simulink library "tqd"  (R2021b)
settings: Solver=VariableStepAuto  StartTime=0.0  StopTime=10.0  RelTol=1e-3
undefined symbols (not defined in the file or in its folder): ATQD_APSDecReq_X_kph, ATQD_APSDecReq_Y_mps2, ATQD_APSDecReqCMD_X_kph, ATQD_APSDecReqTs_X_pct, ATQD_APSDecTimeGain_X_Deg, ATQD_APSDecTimeGain_Y_s, ATQD_APSReqLowSpd_X_Deg, ATQD_AutoHoldReleaseBPS_X_Deg, ATQD_AWDLoadTrqnsGain_X_kg, ATQD_AWDLoadTrqnsGain_Y_pct, ATQD_BOSEnBPSPosn_X_kph, ATQD_BOSMap_X_rpm, ATQD_BOSMap_Y_pct, ATQD_CreepBaseTqD_X_kph, ATQD_CreepBaseTqD_Y_Deg, ATQD_CreepBaseTqR_X_kph, ATQD_CreepBaseTqR_Y_Deg, ATQD_CreepBPSDisPosn_X_Deg, ATQD_CreepBPSDisPosnR_X_Deg, ATQD_CreepBPSEnPosn_X_Deg, ATQD_CreepBPSEnPosnR_X_Deg, ATQD_CreepDeltaTq_X_kph, ATQD_CreepIterm_X_kph, ATQD_CreepIterm_Y_kph, ATQD_CreepItermMaxLimit_X_pct, ATQD_CreepPreloadTime_X_kph, ATQD_CreepPreloadTq_X_kph, ATQD_CreepPreloadTq_Y_s, ATQD_CreepProtTq_X_Deg, ATQD_CreepPterm_X_kph, ATQD_ECOTqMapD_X_rpm, ATQD_ECOTqMapD_Y_pct, ATQD_EOPDTqMapDCon_X_rpm, ATQD_EOPDTqMapDCon_Y_Deg, ATQD_EstInitVehWeight_X_c, ATQD_LHMRollGenMapD_X_rpm, ATQD_LHMRollGenMapD_Y_rpm, ATQD_LHMTqMapD_X_rpm, ATQD_LHMTqMapD_Y_pct, ATQD_NL1TqMapD_X_rpm, ATQD_NL1TqMapD_Y_pct, ATQD_NOPDTqMapDCon_X_rpm, ATQD_NOPDTqMapDCon_Y_Deg, ATQD_NRMRrEDUSpRat_X_rpm, ATQD_NRMRrEDUSpRat_Y_Nm, ATQD_OPDHoldDownRelDelay_X_Deg, ATQD_OPDHoldEnSpd_X_Deg, ATQD_OPDHoldRelDetTime_X_Deg, ATQD_OPDHoldReleaseTq_X_Deg, ATQD_OrigPedTqLowLim_X_Deg, ATQD_OrigPedTqLowLim_Y_pct, ATQD_PedalMapClimbUpLim_X_rpm, ATQD_PedalMapClimbUpLim_Y_Deg, ATQD_PreLoadTq_X_s, ATQD_RollGenMapEL1_X_rpm, ATQD_RollGenMapEL1_Y_rpm, ATQD_SL1TqMapD_X_rpm, ATQD_SL1TqMapD_Y_pct, ATQD_SlideRegenTqGain_X_Gps, ATQD_SlideRegenTqGain_Y_pct ... (+378)
libraries: hcu_lib x59, simulink x49
(part 1 of 12)
settings Model: Creator=13615  LastModifiedBy=FVT22063
settings SolverCC: AlgebraicLoopSolver=TrustRegion
settings DataIOCC: SaveFormat=Array  SignalLoggingSaveFormat=ModelDataLogs  ReturnWorkspaceOutputs=off
settings OptimizationCC: BlockReduction=off  BooleanDataType=off
settings DebuggingCC: SaveWithParameterizedLinksMsg=none  UnderspecifiedInitializationDetection=Classic  MergeDetectMultiDrivingBlocksExec=none  SignalResolutionControl=TryResolveAllWithWarning
settings HardwareCC: TargetUnknown=on
settings ModelReferenceCC: PropagateSignalLabelsOutOfModel=off
settings SFSimCC: SimUseLocalCustomCode=off
settings RTWCC: RTWUseLocalCustomCode=off
settings ConfigComp: CovMetricSettings=dw  CovSaveCumulativeToWorkspaceVar=on  CovSaveSingleToWorkspaceVar=on

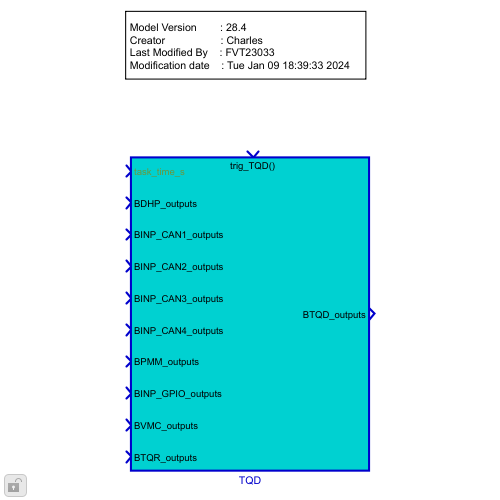
[thumbnail: Simulink's stored preview of the top-level diagram]
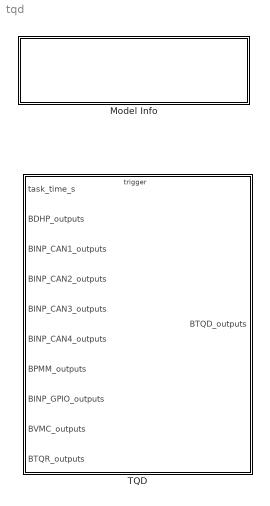
== system tqd ==
  Model Info : Subsystem  LoadFcn=slcm LoadBlock;  InitFcn=slcm('UpdateAllCMBlocksInThisModelInit')  mask(CMBlock){InitialSaveTempField=, InitialBlockCM=None, BlockCM=None, Frame=on, SaveTempField=, DisplayStringWithTags=|, MaskDisplayString=Model Version        : 26.218\nCreator                   : Charles\nLast Modified By    : FVT22063\nModification date    : Thu Sep 19 13:30:35 2024, HorizontalTextAlignment=Left, LeftAlignmentValue=0.02, SourceBlockDiagram=tqd, TagMaxNumber=20, CMTag1=, CMTag2=, CMTag3=, CMTag4=, CMTag5=, CMTag6=, CMTag7=, CMTag8=, CMTag9=, CMTag10=, CMTag11=, CMTag12=, CMTag13=, CMTag14=, CMTag15=, CMTag16=, CMTag17=, CMTag18=, CMTag19=, CMTag20=}
      mask DisplayStringWithTags=|
      | Model Version        : %<ModelVersion>
      | Creator                   : Charles
      | Last Modified By    : %<LastModifiedBy>
      | Modification date    : %<LastModificationDate>
      mask help: This block allows revision control information to be displayed within the model.
      settings: CopyFcn=slcm CopyBlock;  DeleteFcn=slcm Cancel;  PostSaveFcn=slcm('UpdateAllCMBlocksInThisModel')  NameChangeFcn=slcm Rename;  OpenFcn=slcm
      mask Display: text(str2num(LeftAlignmentValue), 0.5, MaskDisplayString, 'HorizontalAlignment', HorizontalTextAlignment)
  TQD : Subsystem
      settings: RTWSystemCode=Nonreusable function  RTWFcnNameOpts=Use subsystem name  RTWFileNameOpts=Use subsystem name

== system tqd/Model Info ==
  EmptySubsystem : Subsystem

== system tqd/TQD ==
  task_time_s : Inport
  BDHP_outputs : Inport  Port=2  OutDataTypeStr=Bus: BDHP_outputs
  BINP_CAN1_outputs : Inport  Port=3  OutDataTypeStr=Bus: BINP_CAN1_outputs
  BINP_CAN2_outputs : Inport  Port=4  OutDataTypeStr=Bus: BINP_CAN2_outputs
  BINP_CAN3_outputs : Inport  Port=5  OutDataTypeStr=Bus: BINP_CAN3_outputs
  BINP_CAN4_outputs : Inport  Port=6  OutDataTypeStr=Bus: BINP_CAN4_outputs
  BPMM_outputs : Inport  Port=7  OutDataTypeStr=Bus: BPMM_outputs
  BINP_GPIO_outputs : Inport  Port=8  OutDataTypeStr=Bus: BINP_GPIO_outputs
  BVMC_outputs : Inport  Port=9  OutDataTypeStr=Bus: BVMC_outputs
  BTQR_outputs : Inport  Port=10  OutDataTypeStr=Bus: BTQR_outputs  LockScale=on
  trig_TQD : TriggerPort  TriggerType=function-call  VariantControl=(inherit)
  Bus Creator1 : BusCreator  Inputs=78  OutDataTypeStr=Bus: BTQD_outputs  NonVirtualBus=on
  Bus Selector : BusSelector  OutputSignals=VINP_IVIPWModeReq_enum,VINP_IVICreepSWReq_flg,VINP_RollModeSWCmd_enum,VINP_IVIPwrLockSW_enum
  Bus Selector1 : BusSelector  OutputSignals=VDHP_ActAPSPosn_pct,VDHP_LowIdleAccPedal_flg
  Bus Selector2 : BusSelector  OutputSignals=VINP_VehSpeed_kph,VINP_BrkSwSta_flg,VINP_BrkSwV_flg,VINP_BrkPedalPos_pct,VINP_BrkPedalPosSta_flg,VINP_FrPTCSActive_flg,VINP_RrPTCSActive_flg,VINP_FrntAxlTrqReqDrv_Nm,VINP_RearAxlTrqReqDrv_Nm,VINP_FrRBCActive_flg,VINP_RrRBCActive_flg,VINP_FrntAxlTrqReqBrk_Nm,VINP_RearAxlTrqReqBrk_Nm,VINP_ADASForceIdle_flg,VINP_CrashOutputSts_enum,VINP_LongAccel_Gps,VINP_EPBCarWashMode_flg,VINP_EPBErrSta_enum,VINP_EPBSta_enum,VINP_DOASta_flg,VINP_HSAActive_flg,VINP_DriverSeatBeltCmd_flg,VINP_AVHActive_flg,VINP_ACCRequiredAccel_mps2,VINP_ACCVehHoldReq_flg,VINP_PsngrSeatBeltCmd_flg,VINP_RDriverSeatBeltCmd_flg,VINP_RCenterSeatBeltCmd_flg,VINP_RPsngrSeatBeltCmd_flg,VINP_SASAngle_Deg,VINP_YawRate_degps,VINP_ADASACCSta_enum,VINP_ABSActive_flg,VINP_ESCActive_flg
  Bus Selector3 : BusSelector  OutputSignals=VINP_BrakeSWGPIO_flg,VINP_CrashSignalGPIO_flg,VINP_DrDoorSW_flg,VINP_SeatSW_flg,VINP_HoodSW_flg,VINP_TailgateSW_flg,VINP_PsDoorSW_flg,VINP_RRDoorSW_flg,VINP_RLDoorSW_flg
  Bus Selector4 : BusSelector  OutputSignals=VINP_ShifterHandleCmd_enum,VINP_FrEDURotateDirction_enum,VINP_RrEDURotateDirction_enum,VINP_FrTMSpd_rpm,VINP_RrTMSpd_rpm,VINP_HVBPwrAvailDchrg_kW,VINP_HVBPwrAvailChrg_kW,VINP_FrRegenAvailTq_Nm,VINP_RrRegenAvailTq_Nm,VINP_FrEDURealTMTq_Nm,VINP_RrEDURealTMTq_Nm,VINP_HVBattErr_flg,VINP_DCDCFaultSta_enum,VINP_FrMotorAvailTq_Nm,VINP_RrMotorAvailTq_Nm,VINP_MCUWarnF_enum,VINP_MCUWarnR_enum,VINP_ChrgPlugSta_enum,VINP_HVBattSOC_pct
  Bus Selector5 : BusSelector  OutputSignals=VVMC_ADASActive_flg,VVMC_ADASWhlTqReq_Nm,VVMC_CruzActive_flg,VVMC_CruzWhlTqReq_Nm,VVMC_MSAActive_flg,VVMC_MSAWhlTqReq_Nm,VVMC_APSActive_flg,VVMC_APSSpeedCMD_kph,VVMC_APSShiftPosnReq_enum,VVMC_ACCPedalOvrd_flg,VVMC_LongAcc_Gps,VVMC_ActMaxSlideRate_pct,VVMC_EstSlope_Deg,VVMC_APSReq_enum,VVMC_RWDRDCActive_enum,VVMC_ActLRSlideRate_pct,VVMC_ActRRSlideRate_pct,VVMC_ActStESCYaw_Dps,VVMC_CAASActive_flg,VVMC_CalibratedGyroY_Dps
  Bus Selector6 : BusSelector  OutputSignals=VINP_RegenMode_enum,VINP_DrSCPSysErrLmp_flg
  Bus Selector7 : BusSelector  OutputSignals=VPMM_PowerSta_enum,VPMM_DrivetrainSelect_enum,VPMM_SysPowerMode_enum
  Bus Selector8 : BusSelector  OutputSignals=VTQR_ActualFEDUWhlTqReq_Nm,VTQR_ActualREDUWhlTqReq_Nm,VTQR_NoABSFEDUWhlTqReq_Nm,VTQR_NoABSREDUWhlTqReq_Nm
  Ground{,1,3..4} (4 alike) : Ground
  TorqueDemand : Subsystem
  BTQD_outputs : Outport  OutDataTypeStr=Bus: BTQD_outputs
  wires:
  Bus Selector2/20 -> TorqueDemand/26(VINP_DOASta_flg)  "<VINP_DOASta_flg>"
  Bus Selector2/19 -> TorqueDemand/25(VINP_EPBSta_enum)  "<VINP_EPBSta_enum>"
  Bus Selector2/18 -> TorqueDemand/24(VINP_EPBErrSta_enum)  "<VINP_EPBErrSta_enum>"
  Bus Selector2/17 -> TorqueDemand/23(VINP_EPBCarWashMode_flg)  "<VINP_EPBCarWashMode_flg>"
  Bus Selector8/2 -> TorqueDemand/97(VTQR_ActualREDUWhlTqReq_Nm)  "<VTQR_ActualREDUWhlTqReq_Nm>"
  Bus Selector2/16 -> TorqueDemand/22(VINP_LongAccel_Gps)  "<VINP_LongAccel_Gps>"
  Bus Selector8/1 -> TorqueDemand/96(VTQR_ActualFEDUWhlTqReq_Nm)  "<VTQR_ActualFEDUWhlTqReq_Nm>"
  Bus Selector5/3 -> TorqueDemand/69(VVMC_CruzActive_flg)  "<VVMC_CruzActive_flg>"
  BTQR_outputs/1 -> Bus Selector8/1
  Bus Selector3/2 -> TorqueDemand/88(VINP_CrashSignalGPIO_flg)  "<VINP_CrashSignalGPIO_flg>"
  Bus Selector3/1 -> TorqueDemand/87(VINP_BrakeSWGPIO_flg)  "<VINP_BrakeSWGPIO_flg>"
  Bus Selector5/6 -> TorqueDemand/72(VVMC_MSAWhlTqReq_Nm)  "<VVMC_MSAWhlTqReq_Nm>"
  Bus Selector5/1 -> TorqueDemand/67(VVMC_ADASActive_flg)  "<VVMC_ADASActive_flg>"
  Bus Selector5/5 -> TorqueDemand/71(VVMC_MSAActive_flg)  "<VVMC_MSAActive_flg>"
  Bus Selector5/4 -> TorqueDemand/70(VVMC_CruzWhlTqReq_Nm)  "<VVMC_CruzWhlTqReq_Nm>"
  Bus Selector5/2 -> TorqueDemand/68(VVMC_ADASWhlTqReq_Nm)  "<VVMC_ADASWhlTqReq_Nm>"
  Bus Selector6/1 -> TorqueDemand/64(VINP_RegenMode_enum)  "<VINP_RegenMode_enum>"
  Bus Selector4/13 -> TorqueDemand/57(VINP_DCDCFaultSta_enum)  "<VINP_DCDCFaultSta_enum>"
  Bus Selector4/12 -> TorqueDemand/56(VINP_HVBattErr_flg)  "<VINP_HVBattErr_flg>"
  Bus Selector4/11 -> TorqueDemand/55(VINP_RrEDURealTMTq_Nm)  "<VINP_RrEDURealTMTq_Nm>"
  Bus Selector4/10 -> TorqueDemand/54(VINP_FrEDURealTMTq_Nm)  "<VINP_FrEDURealTMTq_Nm>"
  Bus Selector4/9 -> TorqueDemand/53(VINP_RrRegenAvailTq_Nm)  "<VINP_RrRegenAvailTq_Nm>"
  TorqueDemand/28(VTQD_RrEDURolRgnTq_Nm) -> Bus Creator1/28
  Bus Selector4/8 -> TorqueDemand/52(VINP_FrRegenAvailTq_Nm)  "<VINP_FrRegenAvailTq_Nm>"
  Bus Selector2/15 -> TorqueDemand/21(VINP_CrashOutputSts_enum)  "<VINP_CrashOutputSts_enum>"
  TorqueDemand/8(VTQD_TqSourceFr_enum) -> Bus Creator1/8
  TorqueDemand/22(VTQD_RrRgnDecrSta_flg) -> Bus Creator1/22
  TorqueDemand/26(VTQD_RrEDUActTq_Nm) -> Bus Creator1/26
  BDHP_outputs/1 -> Bus Selector1/1
  TorqueDemand/30(VTQD_RrEDUSpd_rpm) -> Bus Creator1/30
  TorqueDemand/29(VTQD_FrEDUSpd_rpm) -> Bus Creator1/29
  TorqueDemand/27(VTQD_FrEDURolRgnTq_Nm) -> Bus Creator1/27
  TorqueDemand/25(VTQD_FrEDUActTq_Nm) -> Bus Creator1/25
  TorqueDemand/24(VTQD_DriverWhlTqDemRr_Nm) -> Bus Creator1/24
  TorqueDemand/23(VTQD_DriverWhlTqDemFr_Nm) -> Bus Creator1/23
  TorqueDemand/21(VTQD_FrRgnDecrSta_flg) -> Bus Creator1/21
  TorqueDemand/20(VTQD_RrActvDmpDisabReq_flg) -> Bus Creator1/20
  TorqueDemand/19(VTQD_FrActvDmpDisabReq_flg) -> Bus Creator1/19
  TorqueDemand/18(VTQD_PButtonSta_enum) -> Bus Creator1/18
  TorqueDemand/17(VTQD_ShiftGearPosn_enum) -> Bus Creator1/17
  Bus Selector2/5 -> TorqueDemand/11(VINP_BrkPedalPosSta_flg)  "<VINP_BrkPedalPosSta_flg>"
  TorqueDemand/16(VTQD_EVDriveModeValid_flg) -> Bus Creator1/16
  TorqueDemand/15(VTQD_EVDriveMode_enum) -> Bus Creator1/15
  TorqueDemand/14(VTQD_RollRegenEnable_flg) -> Bus Creator1/14
  TorqueDemand/13(VTQD_LimpHomeAct_flg) -> Bus Creator1/13
  TorqueDemand/12(VTQD_TqTargetShaftSpd_rpm) -> Bus Creator1/12
  TorqueDemand/11(VTQD_RrEDUAvailBrkRgnTq_Nm) -> Bus Creator1/11
  TorqueDemand/10(VTQD_FrEDUAvailBrkRgnTq_Nm) -> Bus Creator1/10
  TorqueDemand/9(VTQD_TqSourceRr_enum) -> Bus Creator1/9
  TorqueDemand/7(VTQD_AfterAvailableTqDemRr_Nm) -> Bus Creator1/7
  TorqueDemand/6(VTQD_AfterAvailableTqDemFr_Nm) -> Bus Creator1/6
  TorqueDemand/5(VTQD_DriverWhlTqDem_Nm) -> Bus Creator1/5
  Bus Selector/1 -> TorqueDemand/41(VINP_IVIPWModeReq_enum)  "<VINP_IVIPWModeReq_enum>"
  TorqueDemand/4(VTQD_PBWUnlockTO_flg) -> Bus Creator1/4
  TorqueDemand/3(VTQD_PBWLockTO_flg) -> Bus Creator1/3
  TorqueDemand/2(VTQD_ParkRequest_flg) -> Bus Creator1/2
  TorqueDemand/1(VTQD_GearActualPosn_enum) -> Bus Creator1/1
  BINP_CAN4_outputs/1 -> Bus Selector6/1  "BINP_CAN4_outputs"
  BINP_CAN2_outputs/1 -> Bus Selector/1  "BINP_CAN2_outputs"
  Ground1/1 -> TorqueDemand/100(VINP_PBWMotorPos_enum)
  Bus Selector2/14 -> TorqueDemand/20(VINP_ADASForceIdle_flg)  "<VINP_ADASForceIdle_flg>"
  BVMC_outputs/1 -> Bus Selector5/1
  Bus Selector2/11 -> TorqueDemand/17(VINP_RrRBCActive_flg)  "<VINP_RrRBCActive_flg>"
  Bus Selector2/7 -> TorqueDemand/13(VINP_RrPTCSActive_flg)  "<VINP_RrPTCSActive_flg>"
  Bus Selector7/2 -> TorqueDemand/5(VPMM_DrivetrainSelect_enum)  "<VPMM_DrivetrainSelect_enum>"
  BINP_GPIO_outputs/1 -> Bus Selector3/1
  Bus Selector1/2 -> TorqueDemand/3(VDHP_LowIdleAccPedal_flg)  "<VDHP_LowIdleAccPedal_flg>"
  Bus Selector1/1 -> TorqueDemand/2(VDHP_ActAPSPosn_pct)  "<VDHP_ActAPSPosn_pct>"
  Bus Selector4/3 -> TorqueDemand/47(VINP_RrEDURotateDirction_enum)  "<VINP_RrEDURotateDirction_enum>"
  Bus Selector4/2 -> TorqueDemand/46(VINP_FrEDURotateDirction_enum)  "<VINP_FrEDURotateDirction_enum>"
  Ground3/1 -> TorqueDemand/102(VINP_CreepSW_flg)
  Ground/1 -> TorqueDemand/101(VDDM_LimpHomeAct_flg)
  Bus Selector4/6 -> TorqueDemand/50(VINP_HVBPwrAvailDchrg_kw)  "<VINP_HVBPwrAvailDchrg_kW>"
  Bus Selector4/7 -> TorqueDemand/51(VINP_HVBPwrAvailChrg_kw)  "<VINP_HVBPwrAvailChrg_kW>"
  Bus Selector4/5 -> TorqueDemand/49(VINP_RrTMSpd_RPM)  "<VINP_RrTMSpd_rpm>"
  Bus Selector4/4 -> TorqueDemand/48(VINP_FrTMSpd_RPM)  "<VINP_FrTMSpd_rpm>"
  Bus Selector4/1 -> TorqueDemand/45(VINP_ShifterHandleCmd_enum)  "<VINP_ShifterHandleCmd_enum>"
  Bus Selector2/10 -> TorqueDemand/16(VINP_FrRBCActive_flg)  "<VINP_FrRBCActive_flg>"
  Bus Selector2/9 -> TorqueDemand/15(VINP_RearAxlTrqReqDrv_Nm)  "<VINP_RearAxlTrqReqDrv_Nm>"
  Bus Selector2/8 -> TorqueDemand/14(VINP_FrntAxlTrqReqDrv_Nm)  "<VINP_FrntAxlTrqReqDrv_Nm>"
  Bus Selector2/13 -> TorqueDemand/19(VINP_RearAxlTrqReqBrk_Nm)  "<VINP_RearAxlTrqReqBrk_Nm>"
  Bus Selector2/12 -> TorqueDemand/18(VINP_FrntAxlTrqReqBrk_Nm)  "<VINP_FrntAxlTrqReqBrk_Nm>"
  Bus Selector2/4 -> TorqueDemand/10(VINP_BrkPedalPos_pct)  "<VINP_BrkPedalPos_pct>"
  Bus Selector2/3 -> TorqueDemand/9(VINP_BrkSwV_flg)  "<VINP_BrkSwV_flg>"
  Bus Selector2/2 -> TorqueDemand/8(VINP_BrkSwSta_flg)  "<VINP_BrkSwSta_flg>"
  Bus Selector2/1 -> TorqueDemand/7(VINP_VehSpeed_kph)  "<VINP_VehSpeed_kph>"
  Bus Selector2/6 -> TorqueDemand/12(VINP_FrPTCSActive_flg)  "<VINP_FrPTCSActive_flg>"
  Bus Selector7/1 -> TorqueDemand/4(VPMM_PowerSta_enum)  "<VPMM_PowerSta_enum>"
  task_time_s/1 -> TorqueDemand/1(task_time_s)  "task_time_s"
  BINP_CAN3_outputs/1 -> Bus Selector4/1
  BINP_CAN1_outputs/1 -> Bus Selector2/1
  BPMM_outputs/1 -> Bus Selector7/1
  Bus Creator1/1 -> BTQD_outputs/1  "BTQD_outputs"
  Bus Selector4/14 -> TorqueDemand/58(VINP_FrMotorAvailTq_Nm)  "<VINP_FrMotorAvailTq_Nm>"
  Bus Selector4/15 -> TorqueDemand/59(VINP_RrMotorAvailTq_Nm)  "<VINP_RrMotorAvailTq_Nm>"
  Bus Selector2/21 -> TorqueDemand/27(VINP_HSAActive_flg)  "<VINP_HSAActive_flg>"
  Bus Selector/2 -> TorqueDemand/42(VINP_IVICreepSWReq_flg)  "<VINP_IVICreepSWReq_flg>"
  Bus Selector2/22 -> TorqueDemand/28(VINP_DriverSeatBeltCmd_flg)  "<VINP_DriverSeatBeltCmd_flg>"
  Bus Selector3/3 -> TorqueDemand/89(VINP_DrDoorSW_flg)  "<VINP_DrDoorSW_flg>"
  Bus Selector4/16 -> TorqueDemand/60(VINP_MCUWarnF_enum)  "<VINP_MCUWarnF_enum>"
  Bus Selector4/17 -> TorqueDemand/61(VINP_MCUWarnR_enum)  "<VINP_MCUWarnR_enum>"
  Bus Selector3/4 -> TorqueDemand/90(VINP_SeatSW_flg)  "<VINP_SeatSW_flg>"
  Bus Selector4/18 -> TorqueDemand/62(VINP_ChrgPlugSta_enum)  "<VINP_ChrgPlugSta_enum>"
  TorqueDemand/32(VTQD_FrEDUAvailBrkRgnTqV_flg) -> Bus Creator1/32
  TorqueDemand/31(VTQD_FrEDUSpdValid_flg) -> Bus Creator1/31
  TorqueDemand/33(VTQD_RrEDUSpdValid_flg) -> Bus Creator1/33
  TorqueDemand/34(VTQD_RrEDUAvailBrkRgnTqV_flg) -> Bus Creator1/34
  TorqueDemand/35(VTQD_RgnAbnorSta_flg) -> Bus Creator1/35
  TorqueDemand/36(VTQD_PTCSPermSta_flg) -> Bus Creator1/36
  TorqueDemand/37(VTQD_FrRgnPermSta_flg) -> Bus Creator1/37
  TorqueDemand/38(VTQD_RrRgnPermSta_flg) -> Bus Creator1/38
  TorqueDemand/39(VTQD_ExternalTqAllow_flg) -> Bus Creator1/39
  TorqueDemand/40(VTQD_FrIdcMin_A) -> Bus Creator1/40
  TorqueDemand/41(VTQD_FrIdcMax_A) -> Bus Creator1/41
  TorqueDemand/42(VTQD_FrUdcMin_V) -> Bus Creator1/42
  TorqueDemand/43(VTQD_FrUdcMax_V) -> Bus Creator1/43
  TorqueDemand/44(VTQD_RrIdcMin_A) -> Bus Creator1/44
  TorqueDemand/45(VTQD_RrIdcMax_A) -> Bus Creator1/45
  TorqueDemand/46(VTQD_RrUdcMin_V) -> Bus Creator1/46
  TorqueDemand/47(VTQD_RrUdcMax_V) -> Bus Creator1/47
  TorqueDemand/48(VTQD_CoordWhlTqDemFr_Nm) -> Bus Creator1/48
  TorqueDemand/49(VTQD_CoordWhlTqDemRr_Nm) -> Bus Creator1/49
  TorqueDemand/50(VTQD_CreepEnable_flg) -> Bus Creator1/50
  TorqueDemand/51(VTQD_CrashDetd_flg) -> Bus Creator1/51
  TorqueDemand/52(VTQD_DiagHCrash_flg) -> Bus Creator1/52
  TorqueDemand/53(VTQD_ReBrakeLPReq_flg) -> Bus Creator1/53
  TorqueDemand/54(VTQD_LoSpdBrkCtrl_flg) -> Bus Creator1/54
  TorqueDemand/55(VTQD_LowIdleAccPedal_flg) -> Bus Creator1/55
  TorqueDemand/56(VTQD_APSStaSys_enum) -> Bus Creator1/56
  TorqueDemand/57(VTQD_APSReq_enum) -> Bus Creator1/57
  TorqueDemand/58(VTQD_APSDecReqA_flg) -> Bus Creator1/58
  TorqueDemand/60(VTQD_ExtShftAllow_flg) -> Bus Creator1/60
  TorqueDemand/61(VTQD_EstVehWeightResult_kg) -> Bus Creator1/61
  TorqueDemand/62(VTQD_BOSEnable_flg) -> Bus Creator1/62
  TorqueDemand/63(VTQD_CreepON_flg) -> Bus Creator1/63
  Bus Selector7/3 -> TorqueDemand/6(VPMM_SysPowerMode_enum)  "<VPMM_SysPowerMode_enum>"
  Bus Selector8/3 -> TorqueDemand/98(VTQR_NoABSFEDUWhlTqReq_Nm)  "<VTQR_NoABSFEDUWhlTqReq_Nm>"
  Bus Selector8/4 -> TorqueDemand/99(VTQR_NoABSREDUWhlTqReq_Nm)  "<VTQR_NoABSREDUWhlTqReq_Nm>"
  TorqueDemand/64(VTQD_PreLoadHold_flg) -> Bus Creator1/64
  TorqueDemand/65(VTQD_PreLoadPreEn_flg) -> Bus Creator1/65
  Bus Selector2/23 -> TorqueDemand/29(VINP_AVHActive_flg)  "<VINP_AVHActive_flg>"
  Bus Selector5/7 -> TorqueDemand/73(VVMC_APSActive_flg)  "<VVMC_APSActive_flg>"
  Bus Selector5/8 -> TorqueDemand/74(VVMC_APSSpeedCMD_kph)  "<VVMC_APSSpeedCMD_kph>"
  Bus Selector5/9 -> TorqueDemand/75(VVMC_APSShiftPosnReq_enum)  "<VVMC_APSShiftPosnReq_enum>"
  TorqueDemand/59(VTQD_APSDecReq_mps2) -> Bus Creator1/59
  Bus Selector2/24 -> TorqueDemand/30(VINP_ACCRequiredAccel_mps2)  "<VINP_ACCRequiredAccel_mps2>"
  TorqueDemand/66(VTQD_CreepPrLoadEnable_flg) -> Bus Creator1/66
  TorqueDemand/67(VTQD_RDCActive_enum) -> Bus Creator1/67
  Bus Selector2/25 -> TorqueDemand/31(VINP_ACCVehHoldReq_flg)  "<VINP_ACCVehHoldReq_flg>"
  Bus Selector5/10 -> TorqueDemand/76(VVMC_ACCPedalOvrd_flg)  "<VVMC_ACCPedalOvrd_flg>"
  TorqueDemand/68(VTQD_EquivAccPedalSWSta_flg) -> Bus Creator1/68
  TorqueDemand/69(VTQD_DriveProtEn_flg) -> Bus Creator1/69
  TorqueDemand/70(VTQD_ActParkRequest_flg) -> Bus Creator1/70
  Bus Selector2/26 -> TorqueDemand/32(VINP_PsngrSeatBeltCmd_flg)  "<VINP_PsngrSeatBeltCmd_flg>"
  Bus Selector2/27 -> TorqueDemand/33(VINP_RDriverSeatBeltCmd_flg)  "<VINP_RDriverSeatBeltCmd_flg>"
  Bus Selector2/28 -> TorqueDemand/34(VINP_RCenterSeatBeltCmd_flg)  "<VINP_RCenterSeatBeltCmd_flg>"
  Bus Selector2/29 -> TorqueDemand/35(VINP_RPsngrSeatBeltCmd_flg)  "<VINP_RPsngrSeatBeltCmd_flg>"
  Bus Selector2/30 -> TorqueDemand/36(VINP_SASAngle_Deg)  "<VINP_SASAngle_Deg>"
  Bus Selector/3 -> TorqueDemand/43(VINP_RollModeSWCmd_enum)  "<VINP_RollModeSWCmd_enum>"
  Bus Selector5/11 -> TorqueDemand/77(VVMC_LongAcc_Gps)  "<VVMC_LongAcc_Gps>"
  Bus Selector5/12 -> TorqueDemand/78(VVMC_ActMaxSlideRate_pct)  "<VVMC_ActMaxSlideRate_pct>"
  Ground4/1 -> TorqueDemand/66(VINP_SCPSystemMode_enum)
  Bus Selector2/31 -> TorqueDemand/37(VINP_YawRate_degps)  "<VINP_YawRate_degps>"
  TorqueDemand/71(VTQD_RegenTqLimitEn_flg) -> Bus Creator1/71
  TorqueDemand/72(VTQD_PedAccTqEn_flg) -> Bus Creator1/72
  Bus Selector5/13 -> TorqueDemand/79(VVMC_EstSlope_Deg)  "<VVMC_EstSlope_Deg>"
  TorqueDemand/73(VTQD_IVIPwrLockSta_enum) -> Bus Creator1/73
  TorqueDemand/74(VTQD_ExtDoorAllow_flg) -> Bus Creator1/74
  Bus Selector3/5 -> TorqueDemand/91(VINP_HoodSW_flg)  "<VINP_HoodSW_flg>"
  Bus Selector3/6 -> TorqueDemand/92(VINP_TailgateSW_flg)  "<VINP_TailgateSW_flg>"
  Bus Selector3/7 -> TorqueDemand/93(VINP_PsDoorSW_flg)  "<VINP_PsDoorSW_flg>"
  Bus Selector3/8 -> TorqueDemand/94(VINP_RRDoorSW_flg)  "<VINP_RRDoorSW_flg>"
  Bus Selector3/9 -> TorqueDemand/95(VINP_RLDoorSW_flg)  "<VINP_RLDoorSW_flg>"
  Bus Selector/4 -> TorqueDemand/44(VINP_IVIPwrLockSW_enum)  "<VINP_IVIPwrLockSW_enum>"
  Bus Selector5/14 -> TorqueDemand/80(VVMC_APSReq_enum)  "<VVMC_APSReq_enum>"
  Bus Selector5/15 -> TorqueDemand/81(VVMC_RWDRDCActive_enum)  "<VVMC_RWDRDCActive_enum>"
  Bus Selector2/32 -> TorqueDemand/38(VINP_ADASACCSta_enum)  "<VINP_ADASACCSta_enum>"
  Bus Selector5/16 -> TorqueDemand/82(VVMC_ActLRSlideRate_pct)  "<VVMC_ActLRSlideRate_pct>"
  Bus Selector5/17 -> TorqueDemand/83(VVMC_ActRRSlideRate_pct)  "<VVMC_ActRRSlideRate_pct>"
  Bus Selector5/18 -> TorqueDemand/84(VVMC_ActStESCYaw_degps)  "<VVMC_ActStESCYaw_Dps>"
  TorqueDemand/75(VTQD_OPDHoldLamp_flg) -> Bus Creator1/75
  Bus Selector4/19 -> TorqueDemand/63(VINP_HVBattSOC_pct)  "<VINP_HVBattSOC_pct>"
  TorqueDemand/76(VTQD_RegenMode_enum) -> Bus Creator1/76
  TorqueDemand/77(VTQD_VehActSpd_kph) -> Bus Creator1/77
  Bus Selector5/19 -> TorqueDemand/85(VVMC_CAASActive_flg)  "<VVMC_CAASActive_flg>"
  Bus Selector5/20 -> TorqueDemand/86(VVMC_CalibratedGyroY_Dps)  "<VVMC_CalibratedGyroY_Dps>"
  TorqueDemand/78(VTQD_CreepBaseTqD_Nm) -> Bus Creator1/78
  Bus Selector2/33 -> TorqueDemand/39(VINP_ABSActive_flg)  "<VINP_ABSActive_flg>"
  Bus Selector2/34 -> TorqueDemand/40(VINP_ESCActive_flg)  "<VINP_ESCActive_flg>"
  Bus Selector6/2 -> TorqueDemand/65(VINP_DrSCPSysErrLmp_enum)  "<VINP_DrSCPSysErrLmp_flg>"

== system tqd/Model Info/EmptySubsystem ==
